simulink model "pendubotSim"  (R2017b)
settings: Solver=FixedStepAuto  StartTime=0.0  StopTime=200  FixedStep=h  RelTol=1e-3  EnableMultiTasking=on
values from neighbouring files (symbols this model uses):
  h = 0.01    [controllerData4.m]
  x0 = [0.55*pi 0.45*pi 0 0]    [controllerData4.m]
undefined symbols (not defined in the file or in its folder): K
libraries: simulink x1
settings Model: Creator=wout  LastModifiedBy=geert
settings SolverCC: ZeroCrossAlgorithm=Adaptive
settings DataIOCC: LimitDataPoints=on
settings OptimizationCC: LifeSpan=inf
settings DebuggingCC: AllowSymbolicDim=off  SFUnexpectedBacktrackingDiag=warning  SFNoUnconditionalDefaultTransitionDiag=warning  SFExecutionAtInitializationDiag=none
settings ModelReferenceCC: PropagateSignalLabelsOutOfModel=off
settings CodeAppCC: StateflowObjectComments=on
settings GRTTargetCC: TargetLangStandard=C89/C90 (ANSI)
settings ConfigComp: CovMetricSettings=dw  CovHtmlReporting=on  CovSaveCumulativeToWorkspaceVar=on  CovSaveSingleToWorkspaceVar=on  CovExternalEMLEnable=off

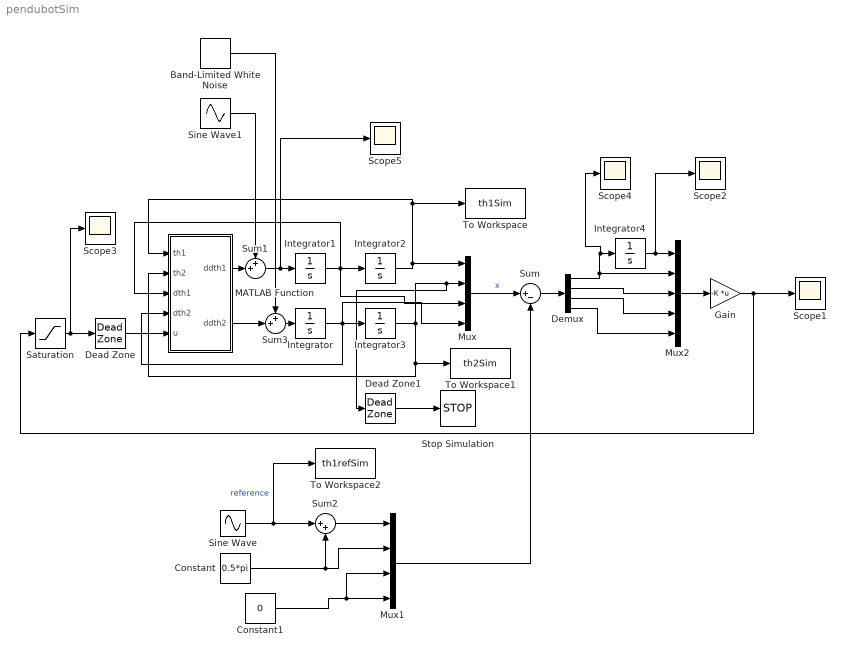
== system pendubotSim ==
  Band-Limited White Noise : simulink/Sources/Band-Limited White Noise  Cov=[2]  Ts=h  seed=[23345]
  Constant : Constant  Value=0.5*pi
  Constant1 : Constant  Value=0
  Dead Zone : DeadZone  LowerValue=-0.3  UpperValue=0.3  SaturateOnIntegerOverflow=on
  Dead Zone1 : DeadZone  LowerValue=0  UpperValue=pi  SaturateOnIntegerOverflow=on
  Demux : Demux
  Gain : Gain  Gain=-K  Multiplication=Matrix(K*u)
  Integrator : Integrator  InitialCondition=x0(4)
  Integrator1 : Integrator  InitialCondition=x0(3)
  Integrator2 : Integrator  InitialCondition=x0(1)  WrapState=on
  Integrator3 : Integrator  InitialCondition=x0(2)  WrapState=on
  Integrator4 : Integrator  LimitOutput=on  UpperSaturationLimit=2  LowerSaturationLimit=-2
  MATLAB Function : MATLAB Function  TreatAsAtomicUnit=on
  Mux : Mux
  Mux1 : Mux
  Mux2 : Mux  Inputs=5
  Saturation : Saturate  UpperLimit=1  LowerLimit=-1
  Scope{1..5} (5 alike) : Scope
  Sine Wave : Sin  Amplitude=0*pi  Frequency=0.1  SampleTime=0
  Sine Wave1 : Sin  Amplitude=5  Frequency=10  SampleTime=0
  Stop Simulation : Stop
  Sum : Sum  Inputs=|+-
  Sum1 : Sum  Inputs=++|
  Sum2 : Sum  Inputs=|++
  Sum3 : Sum  Inputs=++|
  To Workspace : ToWorkspace  VariableName=th1Sim  SampleTime=-1
  To Workspace1 : ToWorkspace  VariableName=th2Sim  SampleTime=-1
  To Workspace2 : ToWorkspace  VariableName=th1refSim  SampleTime=-1
  wires:
  Integrator1/1 -> Mux/3, MATLAB Function/3(dth1), Integrator2/1
  Integrator/1 -> Mux/4, MATLAB Function/4(dth2), Integrator3/1
  Integrator3/1 -> MATLAB Function/2(th2), To Workspace1/1, Mux/2, Dead Zone1/1
  Integrator2/1 -> MATLAB Function/1(th1), To Workspace/1, Mux/1
  Sine Wave/1 -> To Workspace2/1, Sum2/1  "reference"
  Constant/1 -> Mux1/2, Sum2/2
  Sum2/1 -> Mux1/1
  Mux1/1 -> Sum/2
  Sum1/1 -> Scope5/1, Integrator1/1
  MATLAB Function/1(ddth1) -> Sum1/2
  MATLAB Function/2(ddth2) -> Sum3/2
  Sum3/1 -> Integrator/1
  Sine Wave1/1 -> Sum1/1
  Band-Limited White Noise/1 -> Sum3/1
  Saturation/1 -> Scope3/1, Dead Zone/1
  Dead Zone/1 -> MATLAB Function/5(u)
  Dead Zone1/1 -> Stop Simulation/1
  Constant1/1 -> Mux1/3, Mux1/4
  Gain/1 -> Saturation/1, Scope1/1
  Mux/1 -> Sum/1  "x"
  Sum/1 -> Demux/1
  Integrator4/1 -> Scope2/1, Mux2/1
  Mux2/1 -> Gain/1
  Demux/4 -> Mux2/5
  Demux/3 -> Mux2/4
  Demux/2 -> Mux2/3
  Demux/1 -> Scope4/1, Integrator4/1, Mux2/2

== matlab function pendubotSim/MATLAB Function ==
  data: th1 input; ddth1 output; th2 input; dth1 input; dth2 input; ddth2 output; u input
function [ddth1,ddth2] = pendubot(th1,th2,dth1,dth2,u)
%INPUT
% time(t), x(th1,th2,dth1,dth2)
%OUTPUT
% second time-derivative of theta_1(ddth1) and theta_2(ddth2)

% Set params
l1 = 0.1;
g = 9.806; 

m1 = 0.18;
m2 = 0.06;

c1 = 0.06;
c2 = 0.045;
J1 = 0.037;
J2 = 0.00011; 

K = 1.8;
k1 = 0.35;
k2 = 0.00001;

% Set equ's
g11 = m1*c1^2+m2*l1^2+J1;
g21 = m2*l1*c2*cos(th1-th2);
g12 = m2*l1*c2*cos(th1-th2);
g22 = m2*c2^2+J2;
detG = g11*g22-g21*g12; 

V1 = g*cos(th1)*(m1*c1+m2*l1);
V2 = g*c2*m2*cos(th2);
gradV1 = (1/detG)*(g22*V1-g12*V2);
gradV2 = (1/detG)*(g11*V2-g21*V1);

Fth11 = -(1/detG)*g22*(k1*dth1);
Fth12 = (1/detG)*g21*(k1*dth1); 
Fth21 = (1/detG)*g21*k2*dth2;
Fth22 = -(1/detG)*g11*k2*dth2; 
Gam111 = (1/detG)*(0.5*m2^2*l1^2*c2^2*sin(2*(th1-th2)));
Gam122 = -(1/detG)*g22*(m2*l1*c2*sin(th1-th2)); 
Gam211 = (1/detG)*g11*(m2*l1*c2*sin(th1-th2));
Gam222 = -(1/detG)*(0.5*m2^2*l1^2*c2^2*sin(2*(th1-th2)));


Fu1 = 1/detG*g22*K*u;
Fu2 = -1/detG*g12*K*u; 

ddth1 = Fth11+Fth21-Gam111*dth1^2-Gam122*dth2^2+Fu1-gradV1;
ddth2 = Fth12+Fth22-Gam211*dth1^2-Gam222*dth2^2+Fu2-gradV2;
